simulink model "Bota_sriver_simulink"  (R2020b)
settings: Solver=VariableStepAuto  StartTime=0.0  StopTime=inf  RelTol=1e-3
undefined symbols (not defined in the file): serial
libraries: instrumentlib x2
settings Model: Creator=leftk  LastModifiedBy=leftk

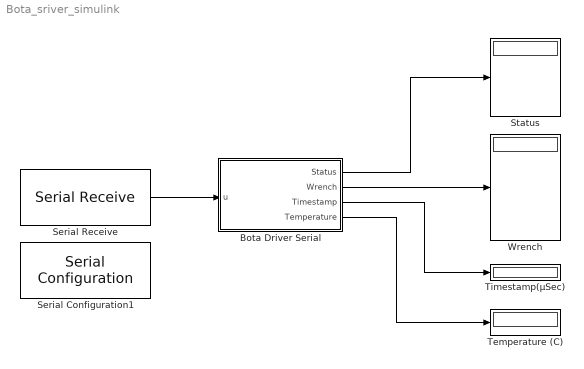
== system Bota_sriver_simulink ==
  Bota Driver Serial : MATLAB Function  TreatAsAtomicUnit=on
  Serial Configuration1 : instrumentlib/Serial Configuration  Priority=-200000  ComPortMenu=COM3  ComPort=COM3  ObjConstructor=serial('COM3');  BaudRate=460800  DataBits=8  Parity=none  StopBits=1  FlowControl=none  Timeout=10  ByteOrder=LittleEndian
  Serial Receive : instrumentlib/Serial Receive  ComPortMenu=COM3  ComPort=COM3  ObjConstructor=serial('COM3');  Header=ª  Terminator=<none>  DataSize="[36   1]"  DataType=uint8  EnableBlockingMode=on  ActionDataUnavailable=Output last received value  CustomValue=0  SampleTime=0.001
  Status : Display
  Temperature (C) : Display
  Timestamp(μSec) : Display
  Wrench : Display
  wires:
  Bota Driver Serial/2(Wrench) -> Wrench/1
  Bota Driver Serial/1(Status) -> Status/1
  Bota Driver Serial/4(Temperature) -> Temperature (C)/1
  Bota Driver Serial/3(Timestamp) -> Timestamp(μSec)/1
  Serial Receive/1 -> Bota Driver Serial/1(u)

== matlab function Bota_sriver_simulink/Bota Driver Serial ==
  data: u input; Status output uint8; Wrench output; Timestamp output uint32; Temperature output single
function [Status, Wrench, Timestamp, Temperature]  = Serial(u)

Timestamp = uint32(0);
Temperature = single(0);
Wrench = zeros(6,1);

Status = de2bi(u(1),4);

Wrench(1) = (typecast(uint8(u(3:6)),'single'));
Wrench(2) = (typecast(uint8(u(7:10)),'single'));
Wrench(3) = (typecast(uint8(u(11:14)),'single'));
Wrench(4) = (typecast(uint8(u(15:18)),'single'));
Wrench(5) = (typecast(uint8(u(19:22)),'single'));
Wrench(6) = (typecast(uint8(u(23:26)),'single'));

Timestamp = (typecast(uint8(u(27:30)),'uint32'));

Temperature = (typecast(uint8(u(31:34)),'single'));

end
